simulink model "SST_MMC"  (R2014a)
settings: Solver=ode45  StartTime=0.0  StopTime=0.2  RelTol=1e-3
libraries: powerlib x328, simulink x1
(part 2 of 3)

== system SST_MMC/MMC_6_SM/arm2/sm4 ==
  " GATE_SIGNAL " : Inport
  " " : powerlib/Measurements/Current Measurement  PhasorSimulation=off  OutputType=Complex  PSBequivalent=0
  " 1" : powerlib/Measurements/Current Measurement  PhasorSimulation=off  OutputType=Complex  PSBequivalent=0
  " 2" : powerlib/Measurements/Current Measurement  PhasorSimulation=off  OutputType=Complex  PSBequivalent=0
  C_SM : powerlib/Elements/Series RLC Branch  LConnTagsString=__new0  RConnTagsString=__new0  BranchType=C  Resistance=1  Inductance=1e-3  SetiL0=off  InitialCurrent=0  Capacitance=C_SM  Setx0=on  InitialVoltage=VC_SM  Measurements=None
  Logical Operator : Logic  Operator=NOT  AllPortsSameDT=off  OutDataTypeStr=boolean
  Mux : Mux  Inputs=2
  Mux1 : Mux  Inputs=2
  VC : powerlib/Measurements/Voltage Measurement  PhasorSimulation=off  OutputType=Complex  PSBequivalent=0
  VC1 : powerlib/Measurements/Voltage Measurement  PhasorSimulation=off  OutputType=Complex  PSBequivalent=0
  VC_GRAPH : Scope
  sw1 : powerlib/Power Electronics/IGBT//Diode  Ron=Ron  Rs=1e5  Cs=inf  Measurements=off
  sw2 : powerlib/Power Electronics/IGBT//Diode  Ron=Ron  Rs=1e5  Cs=inf  Measurements=off
  POSITIVE : PMIOPort  Port=1  Side=Right
  NEGATIVE : PMIOPort  Port=2  Side=Right
  " VC_S_M" : Outport
  " c_ce" : Outport  Port=2
  " smvi" : Outport  Port=3
  wires:
  VC/1 -> " VC_S_M"/1, VC_GRAPH/1
  Logical Operator/1 -> sw1/1
  " GATE_SIGNAL "/1 -> Logical Operator/1, sw2/1
  " 1"/1 -> Mux1/1
  " 2"/1 -> Mux1/2
  " "/1 -> Mux/1
  VC1/1 -> Mux/2
  Mux1/1 -> " c_ce"/1
  Mux/1 -> " smvi"/1
  connections:
  sw1/RConn1 -- " 2"/LConn1
  VC/LConn2 -- C_SM/RConn1 -- sw2/RConn1 -- NEGATIVE/RConn1 -- VC1/LConn2
  VC/LConn1 -- C_SM/LConn1 -- " 1"/RConn1
  POSITIVE/RConn1 -- " "/LConn1 -- VC1/LConn1
  " 1"/LConn1 -- sw1/LConn1
  " 2"/RConn1 -- sw2/LConn1 -- " "/RConn1

== system SST_MMC/MMC_6_SM/arm2/sm5 ==
  " GATE_SIGNAL " : Inport
  " " : powerlib/Measurements/Current Measurement  PhasorSimulation=off  OutputType=Complex  PSBequivalent=0
  " 1" : powerlib/Measurements/Current Measurement  PhasorSimulation=off  OutputType=Complex  PSBequivalent=0
  " 2" : powerlib/Measurements/Current Measurement  PhasorSimulation=off  OutputType=Complex  PSBequivalent=0
  C_SM : powerlib/Elements/Series RLC Branch  LConnTagsString=__new0  RConnTagsString=__new0  BranchType=C  Resistance=1  Inductance=1e-3  SetiL0=off  InitialCurrent=0  Capacitance=C_SM  Setx0=on  InitialVoltage=VC_SM  Measurements=None
  Logical Operator : Logic  Operator=NOT  AllPortsSameDT=off  OutDataTypeStr=boolean
  Mux : Mux  Inputs=2
  Mux1 : Mux  Inputs=2
  VC : powerlib/Measurements/Voltage Measurement  PhasorSimulation=off  OutputType=Complex  PSBequivalent=0
  VC1 : powerlib/Measurements/Voltage Measurement  PhasorSimulation=off  OutputType=Complex  PSBequivalent=0
  VC_GRAPH : Scope
  sw1 : powerlib/Power Electronics/IGBT//Diode  Ron=Ron  Rs=1e5  Cs=inf  Measurements=off
  sw2 : powerlib/Power Electronics/IGBT//Diode  Ron=Ron  Rs=1e5  Cs=inf  Measurements=off
  POSITIVE : PMIOPort  Port=1  Side=Right
  NEGATIVE : PMIOPort  Port=2  Side=Right
  " VC_S_M" : Outport
  " c_ce" : Outport  Port=2
  " smvi" : Outport  Port=3
  wires:
  Mux/1 -> " smvi"/1
  Mux1/1 -> " c_ce"/1
  VC1/1 -> Mux/2
  " "/1 -> Mux/1
  " 2"/1 -> Mux1/2
  " 1"/1 -> Mux1/1
  " GATE_SIGNAL "/1 -> sw2/1, Logical Operator/1
  Logical Operator/1 -> sw1/1
  VC/1 -> VC_GRAPH/1, " VC_S_M"/1
  connections:
  " "/RConn1 -- sw2/LConn1 -- " 2"/RConn1
  " 1"/LConn1 -- sw1/LConn1
  VC1/LConn1 -- " "/LConn1 -- POSITIVE/RConn1
  " 1"/RConn1 -- C_SM/LConn1 -- VC/LConn1
  VC1/LConn2 -- NEGATIVE/RConn1 -- sw2/RConn1 -- C_SM/RConn1 -- VC/LConn2
  sw1/RConn1 -- " 2"/LConn1

== system SST_MMC/MMC_6_SM/arm2/sm6 ==
  " GATE_SIGNAL " : Inport
  " " : powerlib/Measurements/Current Measurement  PhasorSimulation=off  OutputType=Complex  PSBequivalent=0
  " 1" : powerlib/Measurements/Current Measurement  PhasorSimulation=off  OutputType=Complex  PSBequivalent=0
  " 2" : powerlib/Measurements/Current Measurement  PhasorSimulation=off  OutputType=Complex  PSBequivalent=0
  C_SM : powerlib/Elements/Series RLC Branch  LConnTagsString=__new0  RConnTagsString=__new0  BranchType=C  Resistance=1  Inductance=1e-3  SetiL0=off  InitialCurrent=0  Capacitance=C_SM  Setx0=on  InitialVoltage=VC_SM  Measurements=None
  Logical Operator : Logic  Operator=NOT  AllPortsSameDT=off  OutDataTypeStr=boolean
  Mux : Mux  Inputs=2
  Mux1 : Mux  Inputs=2
  VC : powerlib/Measurements/Voltage Measurement  PhasorSimulation=off  OutputType=Complex  PSBequivalent=0
  VC1 : powerlib/Measurements/Voltage Measurement  PhasorSimulation=off  OutputType=Complex  PSBequivalent=0
  VC_GRAPH : Scope
  sw1 : powerlib/Power Electronics/IGBT//Diode  Ron=Ron  Rs=1e5  Cs=inf  Measurements=off
  sw2 : powerlib/Power Electronics/IGBT//Diode  Ron=Ron  Rs=1e5  Cs=inf  Measurements=off
  POSITIVE : PMIOPort  Port=1  Side=Right
  NEGATIVE : PMIOPort  Port=2  Side=Right
  " VC_S_M" : Outport
  " c_ce" : Outport  Port=2
  " smvi" : Outport  Port=3
  wires:
  VC/1 -> " VC_S_M"/1, VC_GRAPH/1
  Logical Operator/1 -> sw1/1
  " GATE_SIGNAL "/1 -> Logical Operator/1, sw2/1
  " 1"/1 -> Mux1/1
  " 2"/1 -> Mux1/2
  " "/1 -> Mux/1
  VC1/1 -> Mux/2
  Mux1/1 -> " c_ce"/1
  Mux/1 -> " smvi"/1
  connections:
  sw1/RConn1 -- " 2"/LConn1
  VC/LConn2 -- C_SM/RConn1 -- sw2/RConn1 -- NEGATIVE/RConn1 -- VC1/LConn2
  VC/LConn1 -- C_SM/LConn1 -- " 1"/RConn1
  POSITIVE/RConn1 -- " "/LConn1 -- VC1/LConn1
  " 1"/LConn1 -- sw1/LConn1
  " 2"/RConn1 -- sw2/LConn1 -- " "/RConn1

== system SST_MMC/MMC_6_SM/arm3/sm1 ==
  " GATE_SIGNAL " : Inport
  " " : powerlib/Measurements/Current Measurement  PhasorSimulation=off  OutputType=Complex  PSBequivalent=0
  " 1" : powerlib/Measurements/Current Measurement  PhasorSimulation=off  OutputType=Complex  PSBequivalent=0
  " 2" : powerlib/Measurements/Current Measurement  PhasorSimulation=off  OutputType=Complex  PSBequivalent=0
  C_SM : powerlib/Elements/Series RLC Branch  LConnTagsString=__new0  RConnTagsString=__new0  BranchType=C  Resistance=1  Inductance=1e-3  SetiL0=off  InitialCurrent=0  Capacitance=C_SM  Setx0=on  InitialVoltage=VC_SM  Measurements=None
  Logical Operator : Logic  Operator=NOT  AllPortsSameDT=off  OutDataTypeStr=boolean
  Mux : Mux  Inputs=2
  Mux1 : Mux  Inputs=2
  VC : powerlib/Measurements/Voltage Measurement  PhasorSimulation=off  OutputType=Complex  PSBequivalent=0
  VC1 : powerlib/Measurements/Voltage Measurement  PhasorSimulation=off  OutputType=Complex  PSBequivalent=0
  VC_GRAPH : Scope
  sw1 : powerlib/Power Electronics/IGBT//Diode  Ron=Ron  Rs=1e5  Cs=inf  Measurements=off
  sw2 : powerlib/Power Electronics/IGBT//Diode  Ron=Ron  Rs=1e5  Cs=inf  Measurements=off
  POSITIVE : PMIOPort  Port=1  Side=Right
  NEGATIVE : PMIOPort  Port=2  Side=Right
  " VC_S_M" : Outport
  " c_ce" : Outport  Port=2
  " smvi" : Outport  Port=3
  wires:
  VC/1 -> " VC_S_M"/1, VC_GRAPH/1
  Logical Operator/1 -> sw1/1
  " GATE_SIGNAL "/1 -> Logical Operator/1, sw2/1
  " 1"/1 -> Mux1/1
  " 2"/1 -> Mux1/2
  " "/1 -> Mux/1
  VC1/1 -> Mux/2
  Mux1/1 -> " c_ce"/1
  Mux/1 -> " smvi"/1
  connections:
  sw1/RConn1 -- " 2"/LConn1
  VC/LConn2 -- C_SM/RConn1 -- sw2/RConn1 -- NEGATIVE/RConn1 -- VC1/LConn2
  VC/LConn1 -- C_SM/LConn1 -- " 1"/RConn1
  POSITIVE/RConn1 -- " "/LConn1 -- VC1/LConn1
  " 1"/LConn1 -- sw1/LConn1
  " 2"/RConn1 -- sw2/LConn1 -- " "/RConn1

== system SST_MMC/MMC_6_SM/arm3/sm2 ==
  " GATE_SIGNAL " : Inport
  " " : powerlib/Measurements/Current Measurement  PhasorSimulation=off  OutputType=Complex  PSBequivalent=0
  " 1" : powerlib/Measurements/Current Measurement  PhasorSimulation=off  OutputType=Complex  PSBequivalent=0
  " 2" : powerlib/Measurements/Current Measurement  PhasorSimulation=off  OutputType=Complex  PSBequivalent=0
  C_SM : powerlib/Elements/Series RLC Branch  LConnTagsString=__new0  RConnTagsString=__new0  BranchType=C  Resistance=1  Inductance=1e-3  SetiL0=off  InitialCurrent=0  Capacitance=C_SM  Setx0=on  InitialVoltage=VC_SM  Measurements=None
  Logical Operator : Logic  Operator=NOT  AllPortsSameDT=off  OutDataTypeStr=boolean
  Mux : Mux  Inputs=2
  Mux1 : Mux  Inputs=2
  VC : powerlib/Measurements/Voltage Measurement  PhasorSimulation=off  OutputType=Complex  PSBequivalent=0
  VC1 : powerlib/Measurements/Voltage Measurement  PhasorSimulation=off  OutputType=Complex  PSBequivalent=0
  VC_GRAPH : Scope
  sw1 : powerlib/Power Electronics/IGBT//Diode  Ron=Ron  Rs=1e5  Cs=inf  Measurements=off
  sw2 : powerlib/Power Electronics/IGBT//Diode  Ron=Ron  Rs=1e5  Cs=inf  Measurements=off
  POSITIVE : PMIOPort  Port=1  Side=Right
  NEGATIVE : PMIOPort  Port=2  Side=Right
  " VC_S_M" : Outport
  " c_ce" : Outport  Port=2
  " smvi" : Outport  Port=3
  wires:
  Mux/1 -> " smvi"/1
  Mux1/1 -> " c_ce"/1
  VC1/1 -> Mux/2
  " "/1 -> Mux/1
  " 2"/1 -> Mux1/2
  " 1"/1 -> Mux1/1
  " GATE_SIGNAL "/1 -> sw2/1, Logical Operator/1
  Logical Operator/1 -> sw1/1
  VC/1 -> VC_GRAPH/1, " VC_S_M"/1
  connections:
  " "/RConn1 -- sw2/LConn1 -- " 2"/RConn1
  " 1"/LConn1 -- sw1/LConn1
  VC1/LConn1 -- " "/LConn1 -- POSITIVE/RConn1
  " 1"/RConn1 -- C_SM/LConn1 -- VC/LConn1
  VC1/LConn2 -- NEGATIVE/RConn1 -- sw2/RConn1 -- C_SM/RConn1 -- VC/LConn2
  sw1/RConn1 -- " 2"/LConn1

== system SST_MMC/MMC_6_SM/arm3/sm3 ==
  " GATE_SIGNAL " : Inport
  " " : powerlib/Measurements/Current Measurement  PhasorSimulation=off  OutputType=Complex  PSBequivalent=0
  " 1" : powerlib/Measurements/Current Measurement  PhasorSimulation=off  OutputType=Complex  PSBequivalent=0
  " 2" : powerlib/Measurements/Current Measurement  PhasorSimulation=off  OutputType=Complex  PSBequivalent=0
  C_SM : powerlib/Elements/Series RLC Branch  LConnTagsString=__new0  RConnTagsString=__new0  BranchType=C  Resistance=1  Inductance=1e-3  SetiL0=off  InitialCurrent=0  Capacitance=C_SM  Setx0=on  InitialVoltage=VC_SM  Measurements=None
  Logical Operator : Logic  Operator=NOT  AllPortsSameDT=off  OutDataTypeStr=boolean
  Mux : Mux  Inputs=2
  Mux1 : Mux  Inputs=2
  VC : powerlib/Measurements/Voltage Measurement  PhasorSimulation=off  OutputType=Complex  PSBequivalent=0
  VC1 : powerlib/Measurements/Voltage Measurement  PhasorSimulation=off  OutputType=Complex  PSBequivalent=0
  VC_GRAPH : Scope
  sw1 : powerlib/Power Electronics/IGBT//Diode  Ron=Ron  Rs=1e5  Cs=inf  Measurements=off
  sw2 : powerlib/Power Electronics/IGBT//Diode  Ron=Ron  Rs=1e5  Cs=inf  Measurements=off
  POSITIVE : PMIOPort  Port=1  Side=Right
  NEGATIVE : PMIOPort  Port=2  Side=Right
  " VC_S_M" : Outport
  " c_ce" : Outport  Port=2
  " smvi" : Outport  Port=3
  wires:
  VC/1 -> " VC_S_M"/1, VC_GRAPH/1
  Logical Operator/1 -> sw1/1
  " GATE_SIGNAL "/1 -> Logical Operator/1, sw2/1
  " 1"/1 -> Mux1/1
  " 2"/1 -> Mux1/2
  " "/1 -> Mux/1
  VC1/1 -> Mux/2
  Mux1/1 -> " c_ce"/1
  Mux/1 -> " smvi"/1
  connections:
  sw1/RConn1 -- " 2"/LConn1
  VC/LConn2 -- C_SM/RConn1 -- sw2/RConn1 -- NEGATIVE/RConn1 -- VC1/LConn2
  VC/LConn1 -- C_SM/LConn1 -- " 1"/RConn1
  POSITIVE/RConn1 -- " "/LConn1 -- VC1/LConn1
  " 1"/LConn1 -- sw1/LConn1
  " 2"/RConn1 -- sw2/LConn1 -- " "/RConn1

== system SST_MMC/MMC_6_SM/arm3/sm4 ==
  " GATE_SIGNAL " : Inport
  " " : powerlib/Measurements/Current Measurement  PhasorSimulation=off  OutputType=Complex  PSBequivalent=0
  " 1" : powerlib/Measurements/Current Measurement  PhasorSimulation=off  OutputType=Complex  PSBequivalent=0
  " 2" : powerlib/Measurements/Current Measurement  PhasorSimulation=off  OutputType=Complex  PSBequivalent=0
  C_SM : powerlib/Elements/Series RLC Branch  LConnTagsString=__new0  RConnTagsString=__new0  BranchType=C  Resistance=1  Inductance=1e-3  SetiL0=off  InitialCurrent=0  Capacitance=C_SM  Setx0=on  InitialVoltage=VC_SM  Measurements=None
  Logical Operator : Logic  Operator=NOT  AllPortsSameDT=off  OutDataTypeStr=boolean
  Mux : Mux  Inputs=2
  Mux1 : Mux  Inputs=2
  VC : powerlib/Measurements/Voltage Measurement  PhasorSimulation=off  OutputType=Complex  PSBequivalent=0
  VC1 : powerlib/Measurements/Voltage Measurement  PhasorSimulation=off  OutputType=Complex  PSBequivalent=0
  VC_GRAPH : Scope
  sw1 : powerlib/Power Electronics/IGBT//Diode  Ron=Ron  Rs=1e5  Cs=inf  Measurements=off
  sw2 : powerlib/Power Electronics/IGBT//Diode  Ron=Ron  Rs=1e5  Cs=inf  Measurements=off
  POSITIVE : PMIOPort  Port=1  Side=Right
  NEGATIVE : PMIOPort  Port=2  Side=Right
  " VC_S_M" : Outport
  " c_ce" : Outport  Port=2
  " smvi" : Outport  Port=3
  wires:
  Mux/1 -> " smvi"/1
  Mux1/1 -> " c_ce"/1
  VC1/1 -> Mux/2
  " "/1 -> Mux/1
  " 2"/1 -> Mux1/2
  " 1"/1 -> Mux1/1
  " GATE_SIGNAL "/1 -> sw2/1, Logical Operator/1
  Logical Operator/1 -> sw1/1
  VC/1 -> VC_GRAPH/1, " VC_S_M"/1
  connections:
  " "/RConn1 -- sw2/LConn1 -- " 2"/RConn1
  " 1"/LConn1 -- sw1/LConn1
  VC1/LConn1 -- " "/LConn1 -- POSITIVE/RConn1
  " 1"/RConn1 -- C_SM/LConn1 -- VC/LConn1
  VC1/LConn2 -- NEGATIVE/RConn1 -- sw2/RConn1 -- C_SM/RConn1 -- VC/LConn2
  sw1/RConn1 -- " 2"/LConn1

== system SST_MMC/MMC_6_SM/arm3/sm5 ==
  " GATE_SIGNAL " : Inport
  " " : powerlib/Measurements/Current Measurement  PhasorSimulation=off  OutputType=Complex  PSBequivalent=0
  " 1" : powerlib/Measurements/Current Measurement  PhasorSimulation=off  OutputType=Complex  PSBequivalent=0
  " 2" : powerlib/Measurements/Current Measurement  PhasorSimulation=off  OutputType=Complex  PSBequivalent=0
  C_SM : powerlib/Elements/Series RLC Branch  LConnTagsString=__new0  RConnTagsString=__new0  BranchType=C  Resistance=1  Inductance=1e-3  SetiL0=off  InitialCurrent=0  Capacitance=C_SM  Setx0=on  InitialVoltage=VC_SM  Measurements=None
  Logical Operator : Logic  Operator=NOT  AllPortsSameDT=off  OutDataTypeStr=boolean
  Mux : Mux  Inputs=2
  Mux1 : Mux  Inputs=2
  VC : powerlib/Measurements/Voltage Measurement  PhasorSimulation=off  OutputType=Complex  PSBequivalent=0
  VC1 : powerlib/Measurements/Voltage Measurement  PhasorSimulation=off  OutputType=Complex  PSBequivalent=0
  VC_GRAPH : Scope
  sw1 : powerlib/Power Electronics/IGBT//Diode  Ron=Ron  Rs=1e5  Cs=inf  Measurements=off
  sw2 : powerlib/Power Electronics/IGBT//Diode  Ron=Ron  Rs=1e5  Cs=inf  Measurements=off
  POSITIVE : PMIOPort  Port=1  Side=Right
  NEGATIVE : PMIOPort  Port=2  Side=Right
  " VC_S_M" : Outport
  " c_ce" : Outport  Port=2
  " smvi" : Outport  Port=3
  wires:
  VC/1 -> " VC_S_M"/1, VC_GRAPH/1
  Logical Operator/1 -> sw1/1
  " GATE_SIGNAL "/1 -> Logical Operator/1, sw2/1
  " 1"/1 -> Mux1/1
  " 2"/1 -> Mux1/2
  " "/1 -> Mux/1
  VC1/1 -> Mux/2
  Mux1/1 -> " c_ce"/1
  Mux/1 -> " smvi"/1
  connections:
  sw1/RConn1 -- " 2"/LConn1
  VC/LConn2 -- C_SM/RConn1 -- sw2/RConn1 -- NEGATIVE/RConn1 -- VC1/LConn2
  VC/LConn1 -- C_SM/LConn1 -- " 1"/RConn1
  POSITIVE/RConn1 -- " "/LConn1 -- VC1/LConn1
  " 1"/LConn1 -- sw1/LConn1
  " 2"/RConn1 -- sw2/LConn1 -- " "/RConn1

== system SST_MMC/MMC_6_SM/arm3/sm6 ==
  " GATE_SIGNAL " : Inport
  " " : powerlib/Measurements/Current Measurement  PhasorSimulation=off  OutputType=Complex  PSBequivalent=0
  " 1" : powerlib/Measurements/Current Measurement  PhasorSimulation=off  OutputType=Complex  PSBequivalent=0
  " 2" : powerlib/Measurements/Current Measurement  PhasorSimulation=off  OutputType=Complex  PSBequivalent=0
  C_SM : powerlib/Elements/Series RLC Branch  LConnTagsString=__new0  RConnTagsString=__new0  BranchType=C  Resistance=1  Inductance=1e-3  SetiL0=off  InitialCurrent=0  Capacitance=C_SM  Setx0=on  InitialVoltage=VC_SM  Measurements=None
  Logical Operator : Logic  Operator=NOT  AllPortsSameDT=off  OutDataTypeStr=boolean
  Mux : Mux  Inputs=2
  Mux1 : Mux  Inputs=2
  VC : powerlib/Measurements/Voltage Measurement  PhasorSimulation=off  OutputType=Complex  PSBequivalent=0
  VC1 : powerlib/Measurements/Voltage Measurement  PhasorSimulation=off  OutputType=Complex  PSBequivalent=0
  VC_GRAPH : Scope
  sw1 : powerlib/Power Electronics/IGBT//Diode  Ron=Ron  Rs=1e5  Cs=inf  Measurements=off
  sw2 : powerlib/Power Electronics/IGBT//Diode  Ron=Ron  Rs=1e5  Cs=inf  Measurements=off
  POSITIVE : PMIOPort  Port=1  Side=Right
  NEGATIVE : PMIOPort  Port=2  Side=Right
  " VC_S_M" : Outport
  " c_ce" : Outport  Port=2
  " smvi" : Outport  Port=3
  wires:
  Mux/1 -> " smvi"/1
  Mux1/1 -> " c_ce"/1
  VC1/1 -> Mux/2
  " "/1 -> Mux/1
  " 2"/1 -> Mux1/2
  " 1"/1 -> Mux1/1
  " GATE_SIGNAL "/1 -> sw2/1, Logical Operator/1
  Logical Operator/1 -> sw1/1
  VC/1 -> VC_GRAPH/1, " VC_S_M"/1
  connections:
  " "/RConn1 -- sw2/LConn1 -- " 2"/RConn1
  " 1"/LConn1 -- sw1/LConn1
  VC1/LConn1 -- " "/LConn1 -- POSITIVE/RConn1
  " 1"/RConn1 -- C_SM/LConn1 -- VC/LConn1
  VC1/LConn2 -- NEGATIVE/RConn1 -- sw2/RConn1 -- C_SM/RConn1 -- VC/LConn2
  sw1/RConn1 -- " 2"/LConn1

== system SST_MMC/MMC_6_SM/arm4/sm1 ==
  " GATE_SIGNAL " : Inport
  " " : powerlib/Measurements/Current Measurement  PhasorSimulation=off  OutputType=Complex  PSBequivalent=0
  " 1" : powerlib/Measurements/Current Measurement  PhasorSimulation=off  OutputType=Complex  PSBequivalent=0
  " 2" : powerlib/Measurements/Current Measurement  PhasorSimulation=off  OutputType=Complex  PSBequivalent=0
  C_SM : powerlib/Elements/Series RLC Branch  LConnTagsString=__new0  RConnTagsString=__new0  BranchType=C  Resistance=1  Inductance=1e-3  SetiL0=off  InitialCurrent=0  Capacitance=C_SM  Setx0=on  InitialVoltage=VC_SM  Measurements=None
  Logical Operator : Logic  Operator=NOT  AllPortsSameDT=off  OutDataTypeStr=boolean
  Mux : Mux  Inputs=2
  Mux1 : Mux  Inputs=2
  VC : powerlib/Measurements/Voltage Measurement  PhasorSimulation=off  OutputType=Complex  PSBequivalent=0
  VC1 : powerlib/Measurements/Voltage Measurement  PhasorSimulation=off  OutputType=Complex  PSBequivalent=0
  VC_GRAPH : Scope
  sw1 : powerlib/Power Electronics/IGBT//Diode  Ron=Ron  Rs=1e5  Cs=inf  Measurements=off
  sw2 : powerlib/Power Electronics/IGBT//Diode  Ron=Ron  Rs=1e5  Cs=inf  Measurements=off
  POSITIVE : PMIOPort  Port=1  Side=Right
  NEGATIVE : PMIOPort  Port=2  Side=Right
  " VC_S_M" : Outport
  " c_ce" : Outport  Port=2
  " smvi" : Outport  Port=3
  wires:
  Mux/1 -> " smvi"/1
  Mux1/1 -> " c_ce"/1
  VC1/1 -> Mux/2
  " "/1 -> Mux/1
  " 2"/1 -> Mux1/2
  " 1"/1 -> Mux1/1
  " GATE_SIGNAL "/1 -> sw2/1, Logical Operator/1
  Logical Operator/1 -> sw1/1
  VC/1 -> VC_GRAPH/1, " VC_S_M"/1
  connections:
  " "/RConn1 -- sw2/LConn1 -- " 2"/RConn1
  " 1"/LConn1 -- sw1/LConn1
  VC1/LConn1 -- " "/LConn1 -- POSITIVE/RConn1
  " 1"/RConn1 -- C_SM/LConn1 -- VC/LConn1
  VC1/LConn2 -- NEGATIVE/RConn1 -- sw2/RConn1 -- C_SM/RConn1 -- VC/LConn2
  sw1/RConn1 -- " 2"/LConn1

== system SST_MMC/MMC_6_SM/arm4/sm2 ==
  " GATE_SIGNAL " : Inport
  " " : powerlib/Measurements/Current Measurement  PhasorSimulation=off  OutputType=Complex  PSBequivalent=0
  " 1" : powerlib/Measurements/Current Measurement  PhasorSimulation=off  OutputType=Complex  PSBequivalent=0
  " 2" : powerlib/Measurements/Current Measurement  PhasorSimulation=off  OutputType=Complex  PSBequivalent=0
  C_SM : powerlib/Elements/Series RLC Branch  LConnTagsString=__new0  RConnTagsString=__new0  BranchType=C  Resistance=1  Inductance=1e-3  SetiL0=off  InitialCurrent=0  Capacitance=C_SM  Setx0=on  InitialVoltage=VC_SM  Measurements=None
  Logical Operator : Logic  Operator=NOT  AllPortsSameDT=off  OutDataTypeStr=boolean
  Mux : Mux  Inputs=2
  Mux1 : Mux  Inputs=2
  VC : powerlib/Measurements/Voltage Measurement  PhasorSimulation=off  OutputType=Complex  PSBequivalent=0
  VC1 : powerlib/Measurements/Voltage Measurement  PhasorSimulation=off  OutputType=Complex  PSBequivalent=0
  VC_GRAPH : Scope
  sw1 : powerlib/Power Electronics/IGBT//Diode  Ron=Ron  Rs=1e5  Cs=inf  Measurements=off
  sw2 : powerlib/Power Electronics/IGBT//Diode  Ron=Ron  Rs=1e5  Cs=inf  Measurements=off
  POSITIVE : PMIOPort  Port=1  Side=Right
  NEGATIVE : PMIOPort  Port=2  Side=Right
  " VC_S_M" : Outport
  " c_ce" : Outport  Port=2
  " smvi" : Outport  Port=3
  wires:
  VC/1 -> " VC_S_M"/1, VC_GRAPH/1
  Logical Operator/1 -> sw1/1
  " GATE_SIGNAL "/1 -> Logical Operator/1, sw2/1
  " 1"/1 -> Mux1/1
  " 2"/1 -> Mux1/2
  " "/1 -> Mux/1
  VC1/1 -> Mux/2
  Mux1/1 -> " c_ce"/1
  Mux/1 -> " smvi"/1
  connections:
  sw1/RConn1 -- " 2"/LConn1
  VC/LConn2 -- C_SM/RConn1 -- sw2/RConn1 -- NEGATIVE/RConn1 -- VC1/LConn2
  VC/LConn1 -- C_SM/LConn1 -- " 1"/RConn1
  POSITIVE/RConn1 -- " "/LConn1 -- VC1/LConn1
  " 1"/LConn1 -- sw1/LConn1
  " 2"/RConn1 -- sw2/LConn1 -- " "/RConn1

== system SST_MMC/MMC_6_SM/arm4/sm3 ==
  " GATE_SIGNAL " : Inport
  " " : powerlib/Measurements/Current Measurement  PhasorSimulation=off  OutputType=Complex  PSBequivalent=0
  " 1" : powerlib/Measurements/Current Measurement  PhasorSimulation=off  OutputType=Complex  PSBequivalent=0
  " 2" : powerlib/Measurements/Current Measurement  PhasorSimulation=off  OutputType=Complex  PSBequivalent=0
  C_SM : powerlib/Elements/Series RLC Branch  LConnTagsString=__new0  RConnTagsString=__new0  BranchType=C  Resistance=1  Inductance=1e-3  SetiL0=off  InitialCurrent=0  Capacitance=C_SM  Setx0=on  InitialVoltage=VC_SM  Measurements=None
  Logical Operator : Logic  Operator=NOT  AllPortsSameDT=off  OutDataTypeStr=boolean
  Mux : Mux  Inputs=2
  Mux1 : Mux  Inputs=2
  VC : powerlib/Measurements/Voltage Measurement  PhasorSimulation=off  OutputType=Complex  PSBequivalent=0
  VC1 : powerlib/Measurements/Voltage Measurement  PhasorSimulation=off  OutputType=Complex  PSBequivalent=0
  VC_GRAPH : Scope
  sw1 : powerlib/Power Electronics/IGBT//Diode  Ron=Ron  Rs=1e5  Cs=inf  Measurements=off
  sw2 : powerlib/Power Electronics/IGBT//Diode  Ron=Ron  Rs=1e5  Cs=inf  Measurements=off
  POSITIVE : PMIOPort  Port=1  Side=Right
  NEGATIVE : PMIOPort  Port=2  Side=Right
  " VC_S_M" : Outport
  " c_ce" : Outport  Port=2
  " smvi" : Outport  Port=3
  wires:
  Mux/1 -> " smvi"/1
  Mux1/1 -> " c_ce"/1
  VC1/1 -> Mux/2
  " "/1 -> Mux/1
  " 2"/1 -> Mux1/2
  " 1"/1 -> Mux1/1
  " GATE_SIGNAL "/1 -> sw2/1, Logical Operator/1
  Logical Operator/1 -> sw1/1
  VC/1 -> VC_GRAPH/1, " VC_S_M"/1
  connections:
  " "/RConn1 -- sw2/LConn1 -- " 2"/RConn1
  " 1"/LConn1 -- sw1/LConn1
  VC1/LConn1 -- " "/LConn1 -- POSITIVE/RConn1
  " 1"/RConn1 -- C_SM/LConn1 -- VC/LConn1
  VC1/LConn2 -- NEGATIVE/RConn1 -- sw2/RConn1 -- C_SM/RConn1 -- VC/LConn2
  sw1/RConn1 -- " 2"/LConn1

== system SST_MMC/MMC_6_SM/arm4/sm4 ==
  " GATE_SIGNAL " : Inport
  " " : powerlib/Measurements/Current Measurement  PhasorSimulation=off  OutputType=Complex  PSBequivalent=0
  " 1" : powerlib/Measurements/Current Measurement  PhasorSimulation=off  OutputType=Complex  PSBequivalent=0
  " 2" : powerlib/Measurements/Current Measurement  PhasorSimulation=off  OutputType=Complex  PSBequivalent=0
  C_SM : powerlib/Elements/Series RLC Branch  LConnTagsString=__new0  RConnTagsString=__new0  BranchType=C  Resistance=1  Inductance=1e-3  SetiL0=off  InitialCurrent=0  Capacitance=C_SM  Setx0=on  InitialVoltage=VC_SM  Measurements=None
  Logical Operator : Logic  Operator=NOT  AllPortsSameDT=off  OutDataTypeStr=boolean
  Mux : Mux  Inputs=2
  Mux1 : Mux  Inputs=2
  VC : powerlib/Measurements/Voltage Measurement  PhasorSimulation=off  OutputType=Complex  PSBequivalent=0
  VC1 : powerlib/Measurements/Voltage Measurement  PhasorSimulation=off  OutputType=Complex  PSBequivalent=0
  VC_GRAPH : Scope
  sw1 : powerlib/Power Electronics/IGBT//Diode  Ron=Ron  Rs=1e5  Cs=inf  Measurements=off
  sw2 : powerlib/Power Electronics/IGBT//Diode  Ron=Ron  Rs=1e5  Cs=inf  Measurements=off
  POSITIVE : PMIOPort  Port=1  Side=Right
  NEGATIVE : PMIOPort  Port=2  Side=Right
  " VC_S_M" : Outport
  " c_ce" : Outport  Port=2
  " smvi" : Outport  Port=3
  wires:
  VC/1 -> " VC_S_M"/1, VC_GRAPH/1
  Logical Operator/1 -> sw1/1
  " GATE_SIGNAL "/1 -> Logical Operator/1, sw2/1
  " 1"/1 -> Mux1/1
  " 2"/1 -> Mux1/2
  " "/1 -> Mux/1
  VC1/1 -> Mux/2
  Mux1/1 -> " c_ce"/1
  Mux/1 -> " smvi"/1
  connections:
  sw1/RConn1 -- " 2"/LConn1
  VC/LConn2 -- C_SM/RConn1 -- sw2/RConn1 -- NEGATIVE/RConn1 -- VC1/LConn2
  VC/LConn1 -- C_SM/LConn1 -- " 1"/RConn1
  POSITIVE/RConn1 -- " "/LConn1 -- VC1/LConn1
  " 1"/LConn1 -- sw1/LConn1
  " 2"/RConn1 -- sw2/LConn1 -- " "/RConn1

== system SST_MMC/MMC_6_SM/arm4/sm5 ==
  " GATE_SIGNAL " : Inport
  " " : powerlib/Measurements/Current Measurement  PhasorSimulation=off  OutputType=Complex  PSBequivalent=0
  " 1" : powerlib/Measurements/Current Measurement  PhasorSimulation=off  OutputType=Complex  PSBequivalent=0
  " 2" : powerlib/Measurements/Current Measurement  PhasorSimulation=off  OutputType=Complex  PSBequivalent=0
  C_SM : powerlib/Elements/Series RLC Branch  LConnTagsString=__new0  RConnTagsString=__new0  BranchType=C  Resistance=1  Inductance=1e-3  SetiL0=off  InitialCurrent=0  Capacitance=C_SM  Setx0=on  InitialVoltage=VC_SM  Measurements=None
  Logical Operator : Logic  Operator=NOT  AllPortsSameDT=off  OutDataTypeStr=boolean
  Mux : Mux  Inputs=2
  Mux1 : Mux  Inputs=2
  VC : powerlib/Measurements/Voltage Measurement  PhasorSimulation=off  OutputType=Complex  PSBequivalent=0
  VC1 : powerlib/Measurements/Voltage Measurement  PhasorSimulation=off  OutputType=Complex  PSBequivalent=0
  VC_GRAPH : Scope
  sw1 : powerlib/Power Electronics/IGBT//Diode  Ron=Ron  Rs=1e5  Cs=inf  Measurements=off
  sw2 : powerlib/Power Electronics/IGBT//Diode  Ron=Ron  Rs=1e5  Cs=inf  Measurements=off
  POSITIVE : PMIOPort  Port=1  Side=Right
  NEGATIVE : PMIOPort  Port=2  Side=Right
  " VC_S_M" : Outport
  " c_ce" : Outport  Port=2
  " smvi" : Outport  Port=3
  wires:
  Mux/1 -> " smvi"/1
  Mux1/1 -> " c_ce"/1
  VC1/1 -> Mux/2
  " "/1 -> Mux/1
  " 2"/1 -> Mux1/2
  " 1"/1 -> Mux1/1
  " GATE_SIGNAL "/1 -> sw2/1, Logical Operator/1
  Logical Operator/1 -> sw1/1
  VC/1 -> VC_GRAPH/1, " VC_S_M"/1
  connections:
  " "/RConn1 -- sw2/LConn1 -- " 2"/RConn1
  " 1"/LConn1 -- sw1/LConn1
  VC1/LConn1 -- " "/LConn1 -- POSITIVE/RConn1
  " 1"/RConn1 -- C_SM/LConn1 -- VC/LConn1
  VC1/LConn2 -- NEGATIVE/RConn1 -- sw2/RConn1 -- C_SM/RConn1 -- VC/LConn2
  sw1/RConn1 -- " 2"/LConn1

== system SST_MMC/MMC_6_SM/arm4/sm6 ==
  " GATE_SIGNAL " : Inport
  " " : powerlib/Measurements/Current Measurement  PhasorSimulation=off  OutputType=Complex  PSBequivalent=0
  " 1" : powerlib/Measurements/Current Measurement  PhasorSimulation=off  OutputType=Complex  PSBequivalent=0
  " 2" : powerlib/Measurements/Current Measurement  PhasorSimulation=off  OutputType=Complex  PSBequivalent=0
  C_SM : powerlib/Elements/Series RLC Branch  LConnTagsString=__new0  RConnTagsString=__new0  BranchType=C  Resistance=1  Inductance=1e-3  SetiL0=off  InitialCurrent=0  Capacitance=C_SM  Setx0=on  InitialVoltage=VC_SM  Measurements=None
  Logical Operator : Logic  Operator=NOT  AllPortsSameDT=off  OutDataTypeStr=boolean
  Mux : Mux  Inputs=2
  Mux1 : Mux  Inputs=2
  VC : powerlib/Measurements/Voltage Measurement  PhasorSimulation=off  OutputType=Complex  PSBequivalent=0
  VC1 : powerlib/Measurements/Voltage Measurement  PhasorSimulation=off  OutputType=Complex  PSBequivalent=0
  VC_GRAPH : Scope
  sw1 : powerlib/Power Electronics/IGBT//Diode  Ron=Ron  Rs=1e5  Cs=inf  Measurements=off
  sw2 : powerlib/Power Electronics/IGBT//Diode  Ron=Ron  Rs=1e5  Cs=inf  Measurements=off
  POSITIVE : PMIOPort  Port=1  Side=Right
  NEGATIVE : PMIOPort  Port=2  Side=Right
  " VC_S_M" : Outport
  " c_ce" : Outport  Port=2
  " smvi" : Outport  Port=3
  wires:
  VC/1 -> " VC_S_M"/1, VC_GRAPH/1
  Logical Operator/1 -> sw1/1
  " GATE_SIGNAL "/1 -> Logical Operator/1, sw2/1
  " 1"/1 -> Mux1/1
  " 2"/1 -> Mux1/2
  " "/1 -> Mux/1
  VC1/1 -> Mux/2
  Mux1/1 -> " c_ce"/1
  Mux/1 -> " smvi"/1
  connections:
  sw1/RConn1 -- " 2"/LConn1
  VC/LConn2 -- C_SM/RConn1 -- sw2/RConn1 -- NEGATIVE/RConn1 -- VC1/LConn2
  VC/LConn1 -- C_SM/LConn1 -- " 1"/RConn1
  POSITIVE/RConn1 -- " "/LConn1 -- VC1/LConn1
  " 1"/LConn1 -- sw1/LConn1
  " 2"/RConn1 -- sw2/LConn1 -- " "/RConn1

== system SST_MMC/MMC_6_SM/arm5/sm1 ==
  " GATE_SIGNAL " : Inport
  " " : powerlib/Measurements/Current Measurement  PhasorSimulation=off  OutputType=Complex  PSBequivalent=0
  " 1" : powerlib/Measurements/Current Measurement  PhasorSimulation=off  OutputType=Complex  PSBequivalent=0
  " 2" : powerlib/Measurements/Current Measurement  PhasorSimulation=off  OutputType=Complex  PSBequivalent=0
  C_SM : powerlib/Elements/Series RLC Branch  LConnTagsString=__new0  RConnTagsString=__new0  BranchType=C  Resistance=1  Inductance=1e-3  SetiL0=off  InitialCurrent=0  Capacitance=C_SM  Setx0=on  InitialVoltage=VC_SM  Measurements=None
  Logical Operator : Logic  Operator=NOT  AllPortsSameDT=off  OutDataTypeStr=boolean
  Mux : Mux  Inputs=2
  Mux1 : Mux  Inputs=2
  VC : powerlib/Measurements/Voltage Measurement  PhasorSimulation=off  OutputType=Complex  PSBequivalent=0
  VC1 : powerlib/Measurements/Voltage Measurement  PhasorSimulation=off  OutputType=Complex  PSBequivalent=0
  VC_GRAPH : Scope
  sw1 : powerlib/Power Electronics/IGBT//Diode  Ron=Ron  Rs=1e5  Cs=inf  Measurements=off
  sw2 : powerlib/Power Electronics/IGBT//Diode  Ron=Ron  Rs=1e5  Cs=inf  Measurements=off
  POSITIVE : PMIOPort  Port=1  Side=Right
  NEGATIVE : PMIOPort  Port=2  Side=Right
  " VC_S_M" : Outport
  " c_ce" : Outport  Port=2
  " smvi" : Outport  Port=3
  wires:
  VC/1 -> " VC_S_M"/1, VC_GRAPH/1
  Logical Operator/1 -> sw1/1
  " GATE_SIGNAL "/1 -> Logical Operator/1, sw2/1
  " 1"/1 -> Mux1/1
  " 2"/1 -> Mux1/2
  " "/1 -> Mux/1
  VC1/1 -> Mux/2
  Mux1/1 -> " c_ce"/1
  Mux/1 -> " smvi"/1
  connections:
  sw1/RConn1 -- " 2"/LConn1
  VC/LConn2 -- C_SM/RConn1 -- sw2/RConn1 -- NEGATIVE/RConn1 -- VC1/LConn2
  VC/LConn1 -- C_SM/LConn1 -- " 1"/RConn1
  POSITIVE/RConn1 -- " "/LConn1 -- VC1/LConn1
  " 1"/LConn1 -- sw1/LConn1
  " 2"/RConn1 -- sw2/LConn1 -- " "/RConn1

== system SST_MMC/MMC_6_SM/arm5/sm2 ==
  " GATE_SIGNAL " : Inport
  " " : powerlib/Measurements/Current Measurement  PhasorSimulation=off  OutputType=Complex  PSBequivalent=0
  " 1" : powerlib/Measurements/Current Measurement  PhasorSimulation=off  OutputType=Complex  PSBequivalent=0
  " 2" : powerlib/Measurements/Current Measurement  PhasorSimulation=off  OutputType=Complex  PSBequivalent=0
  C_SM : powerlib/Elements/Series RLC Branch  LConnTagsString=__new0  RConnTagsString=__new0  BranchType=C  Resistance=1  Inductance=1e-3  SetiL0=off  InitialCurrent=0  Capacitance=C_SM  Setx0=on  InitialVoltage=VC_SM  Measurements=None
  Logical Operator : Logic  Operator=NOT  AllPortsSameDT=off  OutDataTypeStr=boolean
  Mux : Mux  Inputs=2
  Mux1 : Mux  Inputs=2
  VC : powerlib/Measurements/Voltage Measurement  PhasorSimulation=off  OutputType=Complex  PSBequivalent=0
  VC1 : powerlib/Measurements/Voltage Measurement  PhasorSimulation=off  OutputType=Complex  PSBequivalent=0
  VC_GRAPH : Scope
  sw1 : powerlib/Power Electronics/IGBT//Diode  Ron=Ron  Rs=1e5  Cs=inf  Measurements=off
  sw2 : powerlib/Power Electronics/IGBT//Diode  Ron=Ron  Rs=1e5  Cs=inf  Measurements=off
  POSITIVE : PMIOPort  Port=1  Side=Right
  NEGATIVE : PMIOPort  Port=2  Side=Right
  " VC_S_M" : Outport
  " c_ce" : Outport  Port=2
  " smvi" : Outport  Port=3
  wires:
  Mux/1 -> " smvi"/1
  Mux1/1 -> " c_ce"/1
  VC1/1 -> Mux/2
  " "/1 -> Mux/1
  " 2"/1 -> Mux1/2
  " 1"/1 -> Mux1/1
  " GATE_SIGNAL "/1 -> sw2/1, Logical Operator/1
  Logical Operator/1 -> sw1/1
  VC/1 -> VC_GRAPH/1, " VC_S_M"/1
  connections:
  " "/RConn1 -- sw2/LConn1 -- " 2"/RConn1
  " 1"/LConn1 -- sw1/LConn1
  VC1/LConn1 -- " "/LConn1 -- POSITIVE/RConn1
  " 1"/RConn1 -- C_SM/LConn1 -- VC/LConn1
  VC1/LConn2 -- NEGATIVE/RConn1 -- sw2/RConn1 -- C_SM/RConn1 -- VC/LConn2
  sw1/RConn1 -- " 2"/LConn1

== system SST_MMC/MMC_6_SM/arm5/sm3 ==
  " GATE_SIGNAL " : Inport
  " " : powerlib/Measurements/Current Measurement  PhasorSimulation=off  OutputType=Complex  PSBequivalent=0
  " 1" : powerlib/Measurements/Current Measurement  PhasorSimulation=off  OutputType=Complex  PSBequivalent=0
  " 2" : powerlib/Measurements/Current Measurement  PhasorSimulation=off  OutputType=Complex  PSBequivalent=0
  C_SM : powerlib/Elements/Series RLC Branch  LConnTagsString=__new0  RConnTagsString=__new0  BranchType=C  Resistance=1  Inductance=1e-3  SetiL0=off  InitialCurrent=0  Capacitance=C_SM  Setx0=on  InitialVoltage=VC_SM  Measurements=None
  Logical Operator : Logic  Operator=NOT  AllPortsSameDT=off  OutDataTypeStr=boolean
  Mux : Mux  Inputs=2
  Mux1 : Mux  Inputs=2
  VC : powerlib/Measurements/Voltage Measurement  PhasorSimulation=off  OutputType=Complex  PSBequivalent=0
  VC1 : powerlib/Measurements/Voltage Measurement  PhasorSimulation=off  OutputType=Complex  PSBequivalent=0
  VC_GRAPH : Scope
  sw1 : powerlib/Power Electronics/IGBT//Diode  Ron=Ron  Rs=1e5  Cs=inf  Measurements=off
  sw2 : powerlib/Power Electronics/IGBT//Diode  Ron=Ron  Rs=1e5  Cs=inf  Measurements=off
  POSITIVE : PMIOPort  Port=1  Side=Right
  NEGATIVE : PMIOPort  Port=2  Side=Right
  " VC_S_M" : Outport
  " c_ce" : Outport  Port=2
  " smvi" : Outport  Port=3
  wires:
  VC/1 -> " VC_S_M"/1, VC_GRAPH/1
  Logical Operator/1 -> sw1/1
  " GATE_SIGNAL "/1 -> Logical Operator/1, sw2/1
  " 1"/1 -> Mux1/1
  " 2"/1 -> Mux1/2
  " "/1 -> Mux/1
  VC1/1 -> Mux/2
  Mux1/1 -> " c_ce"/1
  Mux/1 -> " smvi"/1
  connections:
  sw1/RConn1 -- " 2"/LConn1
  VC/LConn2 -- C_SM/RConn1 -- sw2/RConn1 -- NEGATIVE/RConn1 -- VC1/LConn2
  VC/LConn1 -- C_SM/LConn1 -- " 1"/RConn1
  POSITIVE/RConn1 -- " "/LConn1 -- VC1/LConn1
  " 1"/LConn1 -- sw1/LConn1
  " 2"/RConn1 -- sw2/LConn1 -- " "/RConn1

== system SST_MMC/MMC_6_SM/arm5/sm4 ==
  " GATE_SIGNAL " : Inport
  " " : powerlib/Measurements/Current Measurement  PhasorSimulation=off  OutputType=Complex  PSBequivalent=0
  " 1" : powerlib/Measurements/Current Measurement  PhasorSimulation=off  OutputType=Complex  PSBequivalent=0
  " 2" : powerlib/Measurements/Current Measurement  PhasorSimulation=off  OutputType=Complex  PSBequivalent=0
  C_SM : powerlib/Elements/Series RLC Branch  LConnTagsString=__new0  RConnTagsString=__new0  BranchType=C  Resistance=1  Inductance=1e-3  SetiL0=off  InitialCurrent=0  Capacitance=C_SM  Setx0=on  InitialVoltage=VC_SM  Measurements=None
  Logical Operator : Logic  Operator=NOT  AllPortsSameDT=off  OutDataTypeStr=boolean
  Mux : Mux  Inputs=2
  Mux1 : Mux  Inputs=2
  VC : powerlib/Measurements/Voltage Measurement  PhasorSimulation=off  OutputType=Complex  PSBequivalent=0
  VC1 : powerlib/Measurements/Voltage Measurement  PhasorSimulation=off  OutputType=Complex  PSBequivalent=0
  VC_GRAPH : Scope
  sw1 : powerlib/Power Electronics/IGBT//Diode  Ron=Ron  Rs=1e5  Cs=inf  Measurements=off
  sw2 : powerlib/Power Electronics/IGBT//Diode  Ron=Ron  Rs=1e5  Cs=inf  Measurements=off
  POSITIVE : PMIOPort  Port=1  Side=Right
  NEGATIVE : PMIOPort  Port=2  Side=Right
  " VC_S_M" : Outport
  " c_ce" : Outport  Port=2
  " smvi" : Outport  Port=3
  wires:
  Mux/1 -> " smvi"/1
  Mux1/1 -> " c_ce"/1
  VC1/1 -> Mux/2
  " "/1 -> Mux/1
  " 2"/1 -> Mux1/2
  " 1"/1 -> Mux1/1
  " GATE_SIGNAL "/1 -> sw2/1, Logical Operator/1
  Logical Operator/1 -> sw1/1
  VC/1 -> VC_GRAPH/1, " VC_S_M"/1
  connections:
  " "/RConn1 -- sw2/LConn1 -- " 2"/RConn1
  " 1"/LConn1 -- sw1/LConn1
  VC1/LConn1 -- " "/LConn1 -- POSITIVE/RConn1
  " 1"/RConn1 -- C_SM/LConn1 -- VC/LConn1
  VC1/LConn2 -- NEGATIVE/RConn1 -- sw2/RConn1 -- C_SM/RConn1 -- VC/LConn2
  sw1/RConn1 -- " 2"/LConn1

== system SST_MMC/MMC_6_SM/arm5/sm5 ==
  " GATE_SIGNAL " : Inport
  " " : powerlib/Measurements/Current Measurement  PhasorSimulation=off  OutputType=Complex  PSBequivalent=0
  " 1" : powerlib/Measurements/Current Measurement  PhasorSimulation=off  OutputType=Complex  PSBequivalent=0
  " 2" : powerlib/Measurements/Current Measurement  PhasorSimulation=off  OutputType=Complex  PSBequivalent=0
  C_SM : powerlib/Elements/Series RLC Branch  LConnTagsString=__new0  RConnTagsString=__new0  BranchType=C  Resistance=1  Inductance=1e-3  SetiL0=off  InitialCurrent=0  Capacitance=C_SM  Setx0=on  InitialVoltage=VC_SM  Measurements=None
  Logical Operator : Logic  Operator=NOT  AllPortsSameDT=off  OutDataTypeStr=boolean
  Mux : Mux  Inputs=2
  Mux1 : Mux  Inputs=2
  VC : powerlib/Measurements/Voltage Measurement  PhasorSimulation=off  OutputType=Complex  PSBequivalent=0
  VC1 : powerlib/Measurements/Voltage Measurement  PhasorSimulation=off  OutputType=Complex  PSBequivalent=0
  VC_GRAPH : Scope
  sw1 : powerlib/Power Electronics/IGBT//Diode  Ron=Ron  Rs=1e5  Cs=inf  Measurements=off
  sw2 : powerlib/Power Electronics/IGBT//Diode  Ron=Ron  Rs=1e5  Cs=inf  Measurements=off
  POSITIVE : PMIOPort  Port=1  Side=Right
  NEGATIVE : PMIOPort  Port=2  Side=Right
  " VC_S_M" : Outport
  " c_ce" : Outport  Port=2
  " smvi" : Outport  Port=3
  wires:
  VC/1 -> " VC_S_M"/1, VC_GRAPH/1
  Logical Operator/1 -> sw1/1
  " GATE_SIGNAL "/1 -> Logical Operator/1, sw2/1
  " 1"/1 -> Mux1/1
  " 2"/1 -> Mux1/2
  " "/1 -> Mux/1
  VC1/1 -> Mux/2
  Mux1/1 -> " c_ce"/1
  Mux/1 -> " smvi"/1
  connections:
  sw1/RConn1 -- " 2"/LConn1
  VC/LConn2 -- C_SM/RConn1 -- sw2/RConn1 -- NEGATIVE/RConn1 -- VC1/LConn2
  VC/LConn1 -- C_SM/LConn1 -- " 1"/RConn1
  POSITIVE/RConn1 -- " "/LConn1 -- VC1/LConn1
  " 1"/LConn1 -- sw1/LConn1
  " 2"/RConn1 -- sw2/LConn1 -- " "/RConn1

== system SST_MMC/MMC_6_SM/arm5/sm6 ==
  " GATE_SIGNAL " : Inport
  " " : powerlib/Measurements/Current Measurement  PhasorSimulation=off  OutputType=Complex  PSBequivalent=0
  " 1" : powerlib/Measurements/Current Measurement  PhasorSimulation=off  OutputType=Complex  PSBequivalent=0
  " 2" : powerlib/Measurements/Current Measurement  PhasorSimulation=off  OutputType=Complex  PSBequivalent=0
  C_SM : powerlib/Elements/Series RLC Branch  LConnTagsString=__new0  RConnTagsString=__new0  BranchType=C  Resistance=1  Inductance=1e-3  SetiL0=off  InitialCurrent=0  Capacitance=C_SM  Setx0=on  InitialVoltage=VC_SM  Measurements=None
  Logical Operator : Logic  Operator=NOT  AllPortsSameDT=off  OutDataTypeStr=boolean
  Mux : Mux  Inputs=2
  Mux1 : Mux  Inputs=2
  VC : powerlib/Measurements/Voltage Measurement  PhasorSimulation=off  OutputType=Complex  PSBequivalent=0
  VC1 : powerlib/Measurements/Voltage Measurement  PhasorSimulation=off  OutputType=Complex  PSBequivalent=0
  VC_GRAPH : Scope
  sw1 : powerlib/Power Electronics/IGBT//Diode  Ron=Ron  Rs=1e5  Cs=inf  Measurements=off
  sw2 : powerlib/Power Electronics/IGBT//Diode  Ron=Ron  Rs=1e5  Cs=inf  Measurements=off
  POSITIVE : PMIOPort  Port=1  Side=Right
  NEGATIVE : PMIOPort  Port=2  Side=Right
  " VC_S_M" : Outport
  " c_ce" : Outport  Port=2
  " smvi" : Outport  Port=3
  wires:
  Mux/1 -> " smvi"/1
  Mux1/1 -> " c_ce"/1
  VC1/1 -> Mux/2
  " "/1 -> Mux/1
  " 2"/1 -> Mux1/2
  " 1"/1 -> Mux1/1
  " GATE_SIGNAL "/1 -> sw2/1, Logical Operator/1
  Logical Operator/1 -> sw1/1
  VC/1 -> VC_GRAPH/1, " VC_S_M"/1
  connections:
  " "/RConn1 -- sw2/LConn1 -- " 2"/RConn1
  " 1"/LConn1 -- sw1/LConn1
  VC1/LConn1 -- " "/LConn1 -- POSITIVE/RConn1
  " 1"/RConn1 -- C_SM/LConn1 -- VC/LConn1
  VC1/LConn2 -- NEGATIVE/RConn1 -- sw2/RConn1 -- C_SM/RConn1 -- VC/LConn2
  sw1/RConn1 -- " 2"/LConn1

== system SST_MMC/MMC_6_SM/arm6/sm1 ==
  " GATE_SIGNAL " : Inport
  " " : powerlib/Measurements/Current Measurement  PhasorSimulation=off  OutputType=Complex  PSBequivalent=0
  " 1" : powerlib/Measurements/Current Measurement  PhasorSimulation=off  OutputType=Complex  PSBequivalent=0
  " 2" : powerlib/Measurements/Current Measurement  PhasorSimulation=off  OutputType=Complex  PSBequivalent=0
  C_SM : powerlib/Elements/Series RLC Branch  LConnTagsString=__new0  RConnTagsString=__new0  BranchType=C  Resistance=1  Inductance=1e-3  SetiL0=off  InitialCurrent=0  Capacitance=C_SM  Setx0=on  InitialVoltage=VC_SM  Measurements=None
  Logical Operator : Logic  Operator=NOT  AllPortsSameDT=off  OutDataTypeStr=boolean
  Mux : Mux  Inputs=2
  Mux1 : Mux  Inputs=2
  VC : powerlib/Measurements/Voltage Measurement  PhasorSimulation=off  OutputType=Complex  PSBequivalent=0
  VC1 : powerlib/Measurements/Voltage Measurement  PhasorSimulation=off  OutputType=Complex  PSBequivalent=0
  VC_GRAPH : Scope
  sw1 : powerlib/Power Electronics/IGBT//Diode  Ron=Ron  Rs=1e5  Cs=inf  Measurements=off
  sw2 : powerlib/Power Electronics/IGBT//Diode  Ron=Ron  Rs=1e5  Cs=inf  Measurements=off
  POSITIVE : PMIOPort  Port=1  Side=Right
  NEGATIVE : PMIOPort  Port=2  Side=Right
  " VC_S_M" : Outport
  " c_ce" : Outport  Port=2
  " smvi" : Outport  Port=3
  wires:
  Mux/1 -> " smvi"/1
  Mux1/1 -> " c_ce"/1
  VC1/1 -> Mux/2
  " "/1 -> Mux/1
  " 2"/1 -> Mux1/2
  " 1"/1 -> Mux1/1
  " GATE_SIGNAL "/1 -> sw2/1, Logical Operator/1
  Logical Operator/1 -> sw1/1
  VC/1 -> VC_GRAPH/1, " VC_S_M"/1
  connections:
  " "/RConn1 -- sw2/LConn1 -- " 2"/RConn1
  " 1"/LConn1 -- sw1/LConn1
  VC1/LConn1 -- " "/LConn1 -- POSITIVE/RConn1
  " 1"/RConn1 -- C_SM/LConn1 -- VC/LConn1
  VC1/LConn2 -- NEGATIVE/RConn1 -- sw2/RConn1 -- C_SM/RConn1 -- VC/LConn2
  sw1/RConn1 -- " 2"/LConn1

== system SST_MMC/MMC_6_SM/arm6/sm2 ==
  " GATE_SIGNAL " : Inport
  " " : powerlib/Measurements/Current Measurement  PhasorSimulation=off  OutputType=Complex  PSBequivalent=0
  " 1" : powerlib/Measurements/Current Measurement  PhasorSimulation=off  OutputType=Complex  PSBequivalent=0
  " 2" : powerlib/Measurements/Current Measurement  PhasorSimulation=off  OutputType=Complex  PSBequivalent=0
  C_SM : powerlib/Elements/Series RLC Branch  LConnTagsString=__new0  RConnTagsString=__new0  BranchType=C  Resistance=1  Inductance=1e-3  SetiL0=off  InitialCurrent=0  Capacitance=C_SM  Setx0=on  InitialVoltage=VC_SM  Measurements=None
  Logical Operator : Logic  Operator=NOT  AllPortsSameDT=off  OutDataTypeStr=boolean
  Mux : Mux  Inputs=2
  Mux1 : Mux  Inputs=2
  VC : powerlib/Measurements/Voltage Measurement  PhasorSimulation=off  OutputType=Complex  PSBequivalent=0
  VC1 : powerlib/Measurements/Voltage Measurement  PhasorSimulation=off  OutputType=Complex  PSBequivalent=0
  VC_GRAPH : Scope
  sw1 : powerlib/Power Electronics/IGBT//Diode  Ron=Ron  Rs=1e5  Cs=inf  Measurements=off
  sw2 : powerlib/Power Electronics/IGBT//Diode  Ron=Ron  Rs=1e5  Cs=inf  Measurements=off
  POSITIVE : PMIOPort  Port=1  Side=Right
  NEGATIVE : PMIOPort  Port=2  Side=Right
  " VC_S_M" : Outport
  " c_ce" : Outport  Port=2
  " smvi" : Outport  Port=3
  wires:
  VC/1 -> " VC_S_M"/1, VC_GRAPH/1
  Logical Operator/1 -> sw1/1
  " GATE_SIGNAL "/1 -> Logical Operator/1, sw2/1
  " 1"/1 -> Mux1/1
  " 2"/1 -> Mux1/2
  " "/1 -> Mux/1
  VC1/1 -> Mux/2
  Mux1/1 -> " c_ce"/1
  Mux/1 -> " smvi"/1
  connections:
  sw1/RConn1 -- " 2"/LConn1
  VC/LConn2 -- C_SM/RConn1 -- sw2/RConn1 -- NEGATIVE/RConn1 -- VC1/LConn2
  VC/LConn1 -- C_SM/LConn1 -- " 1"/RConn1
  POSITIVE/RConn1 -- " "/LConn1 -- VC1/LConn1
  " 1"/LConn1 -- sw1/LConn1
  " 2"/RConn1 -- sw2/LConn1 -- " "/RConn1

== system SST_MMC/MMC_6_SM/arm6/sm3 ==
  " GATE_SIGNAL " : Inport
  " " : powerlib/Measurements/Current Measurement  PhasorSimulation=off  OutputType=Complex  PSBequivalent=0
  " 1" : powerlib/Measurements/Current Measurement  PhasorSimulation=off  OutputType=Complex  PSBequivalent=0
  " 2" : powerlib/Measurements/Current Measurement  PhasorSimulation=off  OutputType=Complex  PSBequivalent=0
  C_SM : powerlib/Elements/Series RLC Branch  LConnTagsString=__new0  RConnTagsString=__new0  BranchType=C  Resistance=1  Inductance=1e-3  SetiL0=off  InitialCurrent=0  Capacitance=C_SM  Setx0=on  InitialVoltage=VC_SM  Measurements=None
  Logical Operator : Logic  Operator=NOT  AllPortsSameDT=off  OutDataTypeStr=boolean
  Mux : Mux  Inputs=2
  Mux1 : Mux  Inputs=2
  VC : powerlib/Measurements/Voltage Measurement  PhasorSimulation=off  OutputType=Complex  PSBequivalent=0
  VC1 : powerlib/Measurements/Voltage Measurement  PhasorSimulation=off  OutputType=Complex  PSBequivalent=0
  VC_GRAPH : Scope
  sw1 : powerlib/Power Electronics/IGBT//Diode  Ron=Ron  Rs=1e5  Cs=inf  Measurements=off
  sw2 : powerlib/Power Electronics/IGBT//Diode  Ron=Ron  Rs=1e5  Cs=inf  Measurements=off
  POSITIVE : PMIOPort  Port=1  Side=Right
  NEGATIVE : PMIOPort  Port=2  Side=Right
  " VC_S_M" : Outport
  " c_ce" : Outport  Port=2
  " smvi" : Outport  Port=3
  wires:
  Mux/1 -> " smvi"/1
  Mux1/1 -> " c_ce"/1
  VC1/1 -> Mux/2
  " "/1 -> Mux/1
  " 2"/1 -> Mux1/2
  " 1"/1 -> Mux1/1
  " GATE_SIGNAL "/1 -> sw2/1, Logical Operator/1
  Logical Operator/1 -> sw1/1
  VC/1 -> VC_GRAPH/1, " VC_S_M"/1
  connections:
  " "/RConn1 -- sw2/LConn1 -- " 2"/RConn1
  " 1"/LConn1 -- sw1/LConn1
  VC1/LConn1 -- " "/LConn1 -- POSITIVE/RConn1
  " 1"/RConn1 -- C_SM/LConn1 -- VC/LConn1
  VC1/LConn2 -- NEGATIVE/RConn1 -- sw2/RConn1 -- C_SM/RConn1 -- VC/LConn2
  sw1/RConn1 -- " 2"/LConn1

== system SST_MMC/MMC_6_SM/arm6/sm4 ==
  " GATE_SIGNAL " : Inport
  " " : powerlib/Measurements/Current Measurement  PhasorSimulation=off  OutputType=Complex  PSBequivalent=0
  " 1" : powerlib/Measurements/Current Measurement  PhasorSimulation=off  OutputType=Complex  PSBequivalent=0
  " 2" : powerlib/Measurements/Current Measurement  PhasorSimulation=off  OutputType=Complex  PSBequivalent=0
  C_SM : powerlib/Elements/Series RLC Branch  LConnTagsString=__new0  RConnTagsString=__new0  BranchType=C  Resistance=1  Inductance=1e-3  SetiL0=off  InitialCurrent=0  Capacitance=C_SM  Setx0=on  InitialVoltage=VC_SM  Measurements=None
  Logical Operator : Logic  Operator=NOT  AllPortsSameDT=off  OutDataTypeStr=boolean
  Mux : Mux  Inputs=2
  Mux1 : Mux  Inputs=2
  VC : powerlib/Measurements/Voltage Measurement  PhasorSimulation=off  OutputType=Complex  PSBequivalent=0
  VC1 : powerlib/Measurements/Voltage Measurement  PhasorSimulation=off  OutputType=Complex  PSBequivalent=0
  VC_GRAPH : Scope
  sw1 : powerlib/Power Electronics/IGBT//Diode  Ron=Ron  Rs=1e5  Cs=inf  Measurements=off
  sw2 : powerlib/Power Electronics/IGBT//Diode  Ron=Ron  Rs=1e5  Cs=inf  Measurements=off
  POSITIVE : PMIOPort  Port=1  Side=Right
  NEGATIVE : PMIOPort  Port=2  Side=Right
  " VC_S_M" : Outport
  " c_ce" : Outport  Port=2
  " smvi" : Outport  Port=3
  wires:
  VC/1 -> " VC_S_M"/1, VC_GRAPH/1
  Logical Operator/1 -> sw1/1
  " GATE_SIGNAL "/1 -> Logical Operator/1, sw2/1
  " 1"/1 -> Mux1/1
  " 2"/1 -> Mux1/2
  " "/1 -> Mux/1
  VC1/1 -> Mux/2
  Mux1/1 -> " c_ce"/1
  Mux/1 -> " smvi"/1
  connections:
  sw1/RConn1 -- " 2"/LConn1
  VC/LConn2 -- C_SM/RConn1 -- sw2/RConn1 -- NEGATIVE/RConn1 -- VC1/LConn2
  VC/LConn1 -- C_SM/LConn1 -- " 1"/RConn1
  POSITIVE/RConn1 -- " "/LConn1 -- VC1/LConn1
  " 1"/LConn1 -- sw1/LConn1
  " 2"/RConn1 -- sw2/LConn1 -- " "/RConn1

== system SST_MMC/MMC_6_SM/arm6/sm5 ==
  " GATE_SIGNAL " : Inport
  " " : powerlib/Measurements/Current Measurement  PhasorSimulation=off  OutputType=Complex  PSBequivalent=0
  " 1" : powerlib/Measurements/Current Measurement  PhasorSimulation=off  OutputType=Complex  PSBequivalent=0
  " 2" : powerlib/Measurements/Current Measurement  PhasorSimulation=off  OutputType=Complex  PSBequivalent=0
  C_SM : powerlib/Elements/Series RLC Branch  LConnTagsString=__new0  RConnTagsString=__new0  BranchType=C  Resistance=1  Inductance=1e-3  SetiL0=off  InitialCurrent=0  Capacitance=C_SM  Setx0=on  InitialVoltage=VC_SM  Measurements=None
  Logical Operator : Logic  Operator=NOT  AllPortsSameDT=off  OutDataTypeStr=boolean
  Mux : Mux  Inputs=2
  Mux1 : Mux  Inputs=2
  VC : powerlib/Measurements/Voltage Measurement  PhasorSimulation=off  OutputType=Complex  PSBequivalent=0
  VC1 : powerlib/Measurements/Voltage Measurement  PhasorSimulation=off  OutputType=Complex  PSBequivalent=0
  VC_GRAPH : Scope
  sw1 : powerlib/Power Electronics/IGBT//Diode  Ron=Ron  Rs=1e5  Cs=inf  Measurements=off
  sw2 : powerlib/Power Electronics/IGBT//Diode  Ron=Ron  Rs=1e5  Cs=inf  Measurements=off
  POSITIVE : PMIOPort  Port=1  Side=Right
  NEGATIVE : PMIOPort  Port=2  Side=Right
  " VC_S_M" : Outport
  " c_ce" : Outport  Port=2
  " smvi" : Outport  Port=3
  wires:
  Mux/1 -> " smvi"/1
  Mux1/1 -> " c_ce"/1
  VC1/1 -> Mux/2
  " "/1 -> Mux/1
  " 2"/1 -> Mux1/2
  " 1"/1 -> Mux1/1
  " GATE_SIGNAL "/1 -> sw2/1, Logical Operator/1
  Logical Operator/1 -> sw1/1
  VC/1 -> VC_GRAPH/1, " VC_S_M"/1
  connections:
  " "/RConn1 -- sw2/LConn1 -- " 2"/RConn1
  " 1"/LConn1 -- sw1/LConn1
  VC1/LConn1 -- " "/LConn1 -- POSITIVE/RConn1
  " 1"/RConn1 -- C_SM/LConn1 -- VC/LConn1
  VC1/LConn2 -- NEGATIVE/RConn1 -- sw2/RConn1 -- C_SM/RConn1 -- VC/LConn2
  sw1/RConn1 -- " 2"/LConn1
